simulink model "INVKinematics"  (R2020a)
settings: Solver=FixedStepAuto  StartTime=0.0  StopTime=t_final  FixedStep=dt  RelTol=1e-3
settings Model: Creator=m2aali  LastModifiedBy=m2aali

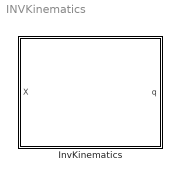
== system INVKinematics ==
  InvKinematics : Subsystem

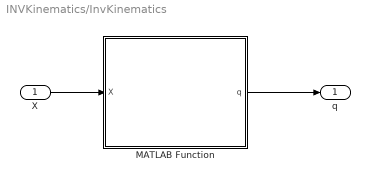
== system INVKinematics/InvKinematics ==
  X : Inport
  MATLAB Function : MATLAB Function  TreatAsAtomicUnit=on
  q : Outport
  wires:
  X/1 -> MATLAB Function/1(X)
  MATLAB Function/1(q) -> q/1

== matlab function INVKinematics/InvKinematics/MATLAB Function ==
  data: X input; q output
function q = INVKinematics(X)
%%% Inverse Kinematic Function
% X is 3*1 vecto of end-effector position in task space, X = [x;y;z]
x = X(1);
y = X(2);
z = X(3);

%% general physical parameters
l1 = 0.6731;
l2 = 0.432;
l3 = 0.434;
lc2 = 0.216;
lc3 = 0.164;

r = sqrt(x^2 + y^2);
R = sqrt(r^2 + (z-l1)^2);
a = atan2(r, z-l1);

%% Inverse Kinematics
% q is 3*1 vector of joint variables (radian), q = [q1;q2;q3]
q1 = atan2(y,x);
q2 = a - atan2(R^2 + l2^2 -l3^2,sqrt(((l2 + l3)^2 - R^2) * (R^2 - (l2 - l3)^2)));
q3 = atan2(R^2 - (l2^2 + l3^2) , sqrt(((l2 + l3)^2 - R^2) * (R^2 - (l2 - l3)^2)));

q = [q1;q2;q3]
